simulink model "deseldetection"  (R2025b)
settings: Solver=VariableStepAuto  StartTime=0.0  StopTime=10  RelTol=1e-3
settings Model: Creator=ujjawalmalani  LastModifiedBy=ujjawalmalani

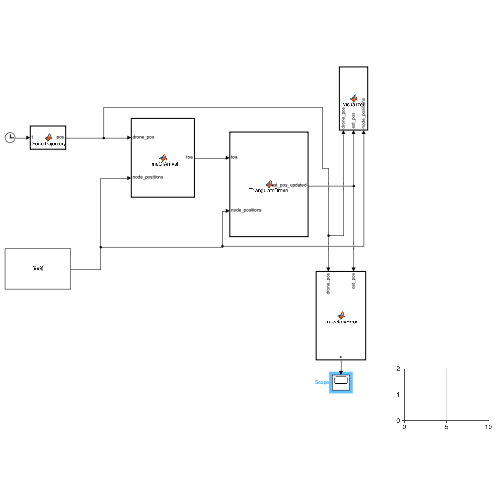
[thumbnail: Simulink's stored preview of the top-level diagram]
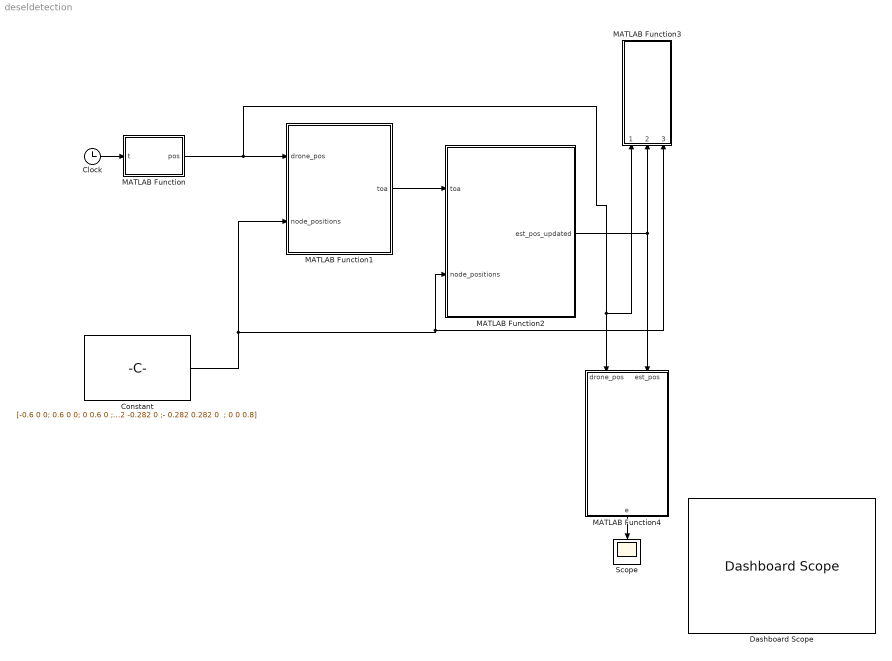
== system deseldetection ==
  Clock : Clock
  Constant : Constant  Value="[-0.6 0 0; 0.6 0 0; 0 0.6 0 ; 0 -0.6 0; 0.282 0.282 0 ; 0.282 -0.282 0 ; -0.282 -0.282 0 ;- 0.282 0.282 0  ; 0 0 0.8]"
  Dashboard Scope : DashboardScope  FontColor=[0.0, 0.0, 0.0]
  MATLAB Function : MATLAB Function  TreatAsAtomicUnit=on
  MATLAB Function1 : MATLAB Function  TreatAsAtomicUnit=on
  MATLAB Function2 : MATLAB Function  TreatAsAtomicUnit=on
  MATLAB Function3 : MATLAB Function  TreatAsAtomicUnit=on
  MATLAB Function4 : MATLAB Function  TreatAsAtomicUnit=on
  Scope : Scope
      settings: ActiveDisplayYMinimum=-0.010937004956854846  ActiveDisplayYMaximum=2.4038074866581294
  wires:
  Clock/1 -> MATLAB Function/1(t)
  Constant/1 -> MATLAB Function1/2(node_positions), MATLAB Function2/2(node_positions), MATLAB Function3/3(node_positions)
  MATLAB Function/1(pos) -> MATLAB Function3/1(drone_pos), MATLAB Function4/1(drone_pos), MATLAB Function1/1(drone_pos)
  MATLAB Function1/1(toa) -> MATLAB Function2/1(toa)
  MATLAB Function2/1(est_pos_updated) -> MATLAB Function4/2(est_pos), MATLAB Function3/2(est_pos)
  MATLAB Function4/1(e) -> Scope/1

== matlab function deseldetection/MATLAB Function1 ==
  data: drone_pos input; toa output; node_positions input
function toa = TimeOfArrival(drone_pos, node_positions)
% TimeOfArrival calculates sound travel time from drone to each sensor node
% drone_pos: [x; y; z] position of drone
% node_positions: 4x3 matrix of node coordinates

c = 343; % Speed of sound in air (m/s)
num_nodes = size(node_positions,1); 
toa = zeros(num_nodes,1); % initialize output

for i = 1:num_nodes
    % distance between drone and node i
    d = norm(drone_pos' - node_positions(i,:)); 
    % time-of-arrival
    toa(i) = d / c;
    
end

end

== matlab function deseldetection/MATLAB Function ==
  data: t input; pos output
function pos = DroneTrajectory(t)
    % Drone 3D trajectory simulation
    R = 10;       % Horizontal radius in meters
    omega = 0.2;  % Angular speed
    x = R*cos(omega*t);
    y = R*sin(omega*t);
    z = 30 + 5*sin(0.5*omega*t); % Altitude oscillation
    pos = [x; y; z]; 
    % Original drone position (meters) 
    noise = 0.5;
    pos = pos + noise*randn(size(pos));

end

== matlab function deseldetection/MATLAB Function2 ==
  data: toa input; est_pos_updated output; node_positions input
function est_pos_updated = TriangulateDrone(toa, node_positions)
% Triangulate drone using TDOA and optionally apply prediction
% Inputs:
%   toa            - Nx1 time-of-arrival measurements
%   node_positions - Nx3 positions of sensor nodes
%   prev_est_pos   - 1x3 previous estimated position (optional)
% Output:
%   est_pos_updated - 1x3 estimated position with prediction

c = 343; % speed of sound
d = toa * c; % convert time to distance

% Node coordinates
x = node_positions(:,1);
y = node_positions(:,2);
z = node_positions(:,3);
prev_est_pos = [0  0  0]; 
prev_est_pos = [prev_est_pos; node_positions];
% Reference node
x1 = x(1); y1 = y(1); z1 = z(1); d1 = d(1);

A = [];
b = [];

for i = 2:length(d)
    A = [A;
         2*(x(i)-x1) 2*(y(i)-y1) 2*(z(i)-z1)];
    b = [b;
        d1^2 - d(i)^2 ...
        - x1^2 + x(i)^2 ...
        - y1^2 + y(i)^2 ...
        - z1^2 + z(i)^2];
end

% Least squares solution (stable)
est_pos = pinv(A)*b;

% Add Gaussian noise
noise_level = 0.5; % meters
est_pos = est_pos + noise_level*randn(size(est_pos));

% --- Prediction / fusion ---
if nargin == 3 && ~isempty(prev_est_pos)
    % Ensure row vectors
    est_pos = est_pos(:)';        % current estimate
    prev_est_pos = prev_est_pos(:)'; % previous estimate

    % Linear velocity prediction
    vel_est = est_pos - prev_est_pos;

    % Predict next position
    pred_pos = est_pos + vel_est;

    % Fuse prediction with current estimate
    alpha = 0.6; % weight for prediction
    est_pos_updated = alpha*pred_pos + (1-alpha)*est_pos;
else
    % First estimate, no prediction
    est_pos_updated = est_pos(:)'; 
end
end

== matlab function deseldetection/MATLAB Function3 ==
  data: drone_pos input; est_pos input; node_positions input
function Visualizer(drone_pos, est_pos, node_positions)

coder.extrinsic('figure','plot3','scatter3','grid','hold','xlabel','ylabel','zlabel','view','drawnow','line')

persistent fig h_nodes h_real_traj h_current_drone h_est_line h_pred_line est_history drone_history

if isempty(fig)
    % Create figure
    fig = figure;
    hold on; grid on; axis equal;
    xlabel('X (m)'); ylabel('Y (m)'); zlabel('Z (m)');
    view(45,30);

    % Plot sensor nodes
    h_nodes = scatter3(node_positions(:,1),node_positions(:,2),node_positions(:,3),80,'yellow','filled');

    % Initialize histories
    drone_history = [];
    est_history   = [];

    % Real drone trajectory (red line)
    h_real_traj = plot3(NaN,NaN,NaN,'r-','LineWidth',2);

    % Current drone position marker (red sphere)
    h_current_drone = scatter3(NaN,NaN,NaN,100,'r','filled');

    % Estimated position line from origin (blue dashed)
    h_est_line = line([0 est_pos(1)],[0 est_pos(2)],[0 est_pos(3)],'Color','b','LineStyle','--','LineWidth',2);

    % Predicted position line from estimated position (magenta dashed)
    h_pred_line = line([NaN NaN],[NaN NaN],[NaN NaN],'Color','m','LineStyle','--','LineWidth',2);

else
    % Append current positions
    drone_history = [drone_history; drone_pos(:)'];
    est_history   = [est_history;   est_pos(:)'];

    % Update real drone trajectory
    set(h_real_traj,'XData',drone_history(:,1),'YData',drone_history(:,2),'ZData',drone_history(:,3));

    % Update current drone marker
    set(h_current_drone,'XData',drone_pos(1),'YData',drone_pos(2),'ZData',drone_pos(3));

    % Update estimated position line from origin
    set(h_est_line,'XData',[0 est_pos(1)],'YData',[0 est_pos(2)],'ZData',[0 est_pos(3)]);

    % Compute simple linear prediction using last two estimated positions
    if size(est_history,1) >= 2
        pos_prev = est_history(end-1,:);
        pos_curr = est_history(end,:);
        vel_est  = pos_curr - pos_prev;        % velocity estimate
        pred_pos = pos_curr + vel_est;         % predicted next position

        % Update prediction line from estimated position to predicted position
        set(h_pred_line,'XData',[pos_curr(1) pred_pos(1)], ...
                        'YData',[pos_curr(2) pred_pos(2)], ...
                        'ZData',[pos_curr(3) pred_pos(3)]);
    end
end

drawnow
end

== matlab function deseldetection/MATLAB Function4 ==
  data: drone_pos input; e output; est_pos input
function e = TrajectoryError(drone_pos, est_pos)
% Euclidean distance error
e = sqrt((drone_pos(1)-est_pos(1))^2 + (drone_pos(2)-est_pos(2))^2  + (drone_pos(3)-est_pos(3))^2);

end
